simulink model "DiffEQsim1"  (Simulink 5.0)
settings: Solver=ode45  StartTime=0.0  StopTime=1  RelTol=1e-3
undefined symbols (not defined in the file or in its folder): sigbuilder_block
settings Model: Creator=mike  LastModifiedBy=mike  ExtModeAutoUpdateStatusClock=off

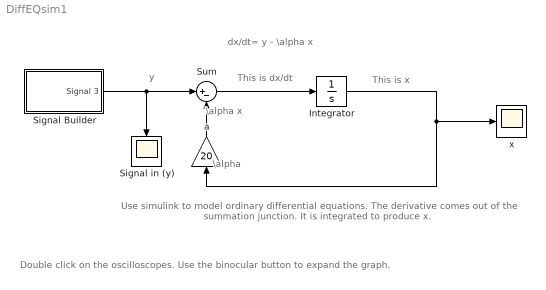
== system DiffEQsim1 ==
  note: This is dx/dt
  note: This is x
  note: dx/dt= y - \alpha x
  note: \alpha
  note: y
  note: \alpha x
  note: Double click on the oscilloscopes. Use the binocular button to expand the graph.
  note: Use simulink to model ordinary differential equations.
      | The derivative comes out of the summation junction.
      | It is integrated to produce x.
  Integrator : Integrator
  Signal Builder : Subsystem  Tag=STV Subsys  StartFcn=sigbuilder_block('start');  StopFcn=sigbuilder_block('stop');  ClipboardFcn=sigbuilder_block('clipboard');  mask(Sigbuilder block){}
      mask help: Sigbuilder GUI
      mask init:
      | if ~strcmp(get_param(bdroot(gcb),'SimulationStatus'),'stopped') tuvar = sigbuilder_block('maskInit'); end
      settings: CopyFcn=sigbuilder_block('copy');  DeleteFcn=sigbuilder_block('delete');  ModelCloseFcn=sigbuilder_block('modelClose');  PreSaveFcn=sigbuilder_block('preSave');  NameChangeFcn=sigbuilder_block('namechange');  OpenFcn=sigbuilder_block('open',[50 50 520 400 ]);  CloseFcn=sigbuilder_block('close');
      mask Display: plot(0,0,100,100,[10,10,40,40,10],[80,20,20,80,80],[40,10],[50,50], [40,27,10],[65,72,56],[40,25,25,10],[28,28,43,43]);
  Signal in (y) : Scope
      settings: Orientation=down  TimeRange=1  YMin=0  YMax=1
  Sum : Sum  Inputs=|+-  SaturateOnIntegerOverflow=on
  a : Gain  Orientation=up  Gain=20  SaturateOnIntegerOverflow=on
  x : Scope
      settings: TimeRange=1  YMin=0  YMax=0.05
  wires:
  Signal Builder/1(Signal 3) -> Sum/1, Signal in (y)/1
  Sum/1 -> Integrator/1
  a/1 -> Sum/2
  Integrator/1 -> a/1, x/1

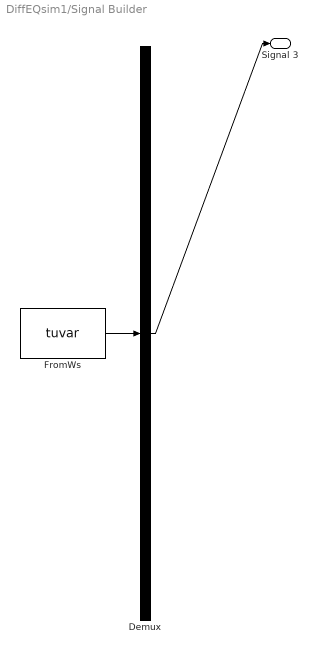
== system DiffEQsim1/Signal Builder ==
  Demux : Demux  Tag=STV Demux  Outputs=1
  FromWs : FromWorkspace  Tag=STV FromWs  VariableName=tuvar  SampleTime=0  SigBuilderData=DataTag0
  Signal 3 : Outport  Tag=STV Outport
  wires:
  FromWs/1 -> Demux/1
  Demux/1 -> Signal 3/1
